simulink model "Oneroom_2015b_Web_Socket"  (R2016a)
settings: Solver=VariableStepAuto  StartTime=0.0  StopTime=Inf  RelTol=1e-3
InitFcn:
  | %server = sim_server(10000);
StartFcn:
  | %The GUI handles are by default hidden, turn them on
  | set(0,'ShowHiddenHandles','on');
  | 
  | %Set up the arguments that will go into the gain block event callback listener
  | blk = 'Oneroom_2015b_Web_Socket/Temperature';
  | event = 'PostOutputs';
  | listener = @updategui;
  | 
  | %Create the listener
  | h = add_exec_event_listener(blk, event, listener);
StopFcn:
  | %server.stop
libraries: simulink x1
settings Model: Creator=accma  LastModifiedBy=e0154145

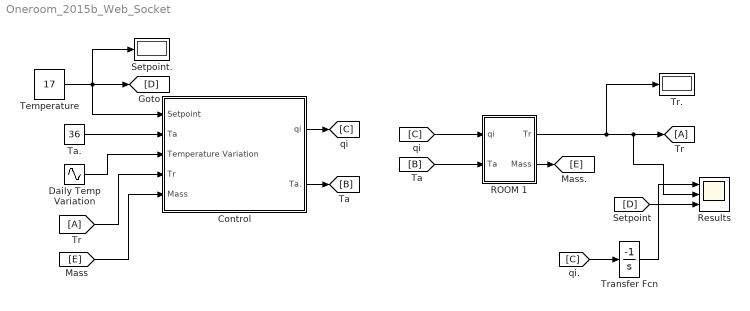
== system Oneroom_2015b_Web_Socket ==
  Control : Subsystem
  Daily Temp Variation : Sin  Amplitude=15  Frequency=2*pi/24  SampleTime=0
  ROOM 1 : Subsystem
  Results : Scope  NumInputPorts=3
  Setpoint. : Display
  Ta. : Constant  Value=36
  Temperature : Constant  Value=17
  Tr. : Display
  Transfer Fcn : TransferFcn  Numerator=[-1]  Denominator=[1 0]
  wires:
  ROOM 1/1(Tr) -> Tr./1, Results/2, [A]
  Ta./1 -> Control/2(Ta)
  Daily Temp Variation/1 -> Control/3(Temperature Variation)
  [B] -> ROOM 1/2(Ta)
  Control/1(qi) -> [C]
  [C] -> ROOM 1/1(qi)
  Control/2(Ta.) -> [B]
  [E] -> Control/5(Mass)
  ROOM 1/2("Mass ") -> [E]
  [A] -> Control/4(Tr)
  [C] -> Transfer Fcn/1
  Transfer Fcn/1 -> Results/1
  [D] -> Results/3
  Temperature/1 -> Control/1(Setpoint), Setpoint./1, [D]

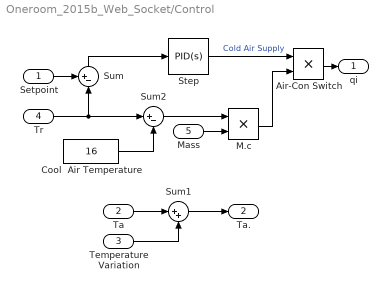
== system Oneroom_2015b_Web_Socket/Control ==
  Setpoint : Inport
  Ta : Inport  Port=2
  Temperature Variation : Inport  Port=3
  Tr : Inport  Port=4
  Mass : Inport  Port=5
  Air-Con Switch : Product  OutMin=16  OutMax=24  RndMeth=Zero
  Cool  Air Temperature : Constant  Value=16
  M.c : Product  RndMeth=Zero
  "Step " : simulink/Continuous/PID Controller  Controller=PID  TimeDomain=Continuous-time  SampleTime=-1  IntegratorMethod=Forward Euler  FilterMethod=Forward Euler  Form=Parallel  UseFilter=on  ControllerParametersSource=internal  P=0.180562771706717  I=1.39450145257241  D=0.00209626055389064  N=23.2260724094918  InitialConditionSource=internal  InitialConditionForIntegrator=0  InitialConditionForFilter=0  ExternalReset=none  LimitOutput=on  UpperSaturationLimit=1  LowerSaturationLimit=-1  LinearizeAsGain=on  AntiWindupMode=none  Kb=1  TrackingMode=off  Kt=1  PParamMin=[]  PParamMax=[]  IParamMin=[]  IParamMax=[]  DParamMin=[]  DParamMax=[]  NParamMin=[]  NParamMax=[]  KbParamMin=[]  KbParamMax=[]  KtParamMin=[]  KtParamMax=[]  POutMin=[]  POutMax=[]  IOutMin=[]  IOutMax=[]  DOutMin=[]  DOutMax=[]  NOutMin=[]  NOutMax=[]  KbOutMin=[]  KbOutMax=[]  KtOutMin=[]  KtOutMax=[]  IntegratorOutMin=[]  IntegratorOutMax=[]  FilterOutMin=[]  FilterOutMax=[]  SumOutMin=[]  SumOutMax=[]  SumI1OutMin=[]  SumI1OutMax=[]  SumI2OutMin=[]  SumI2OutMax=[]  SumI3OutMin=[]  SumI3OutMax=[]  SumDOutMin=[]  SumDOutMax=[]  SaturationOutMin=[]  SaturationOutMax=[]  IntegratorContinuousStateAttributes=''  IntegratorStateMustResolveToSignalObject=off  IntegratorRTWStateStorageClass=Auto  FilterContinuousStateAttributes=''  FilterStateMustResolveToSignalObject=off  FilterRTWStateStorageClass=Auto  DifferentiatorICPrevScaledInput=0  DifferentiatorOutMin=[]  DifferentiatorOutMax=[]
  Sum : Sum  Inputs=+-|  SaturateOnIntegerOverflow=on  InputSameDT=on  OutDataTypeStr=Inherit: Same as first input
  Sum1 : Sum  Inputs=|++  SaturateOnIntegerOverflow=on  InputSameDT=on  OutDataTypeStr=Inherit: Same as first input
  Sum2 : Sum  Inputs=|+-
  qi : Outport
  Ta. : Outport  Port=2
  wires:
  Air-Con Switch/1 -> qi/1
  Ta/1 -> Sum1/1
  Sum1/1 -> Ta./1
  Cool  Air Temperature/1 -> Sum2/2
  Sum/1 -> "Step "/1
  Temperature Variation/1 -> Sum1/2
  Setpoint/1 -> Sum/1
  "Step "/1 -> Air-Con Switch/1  "Cold Air Supply"
  M.c/1 -> Air-Con Switch/2
  Tr/1 -> Sum2/1, Sum/2
  Mass/1 -> M.c/2
  Sum2/1 -> M.c/1

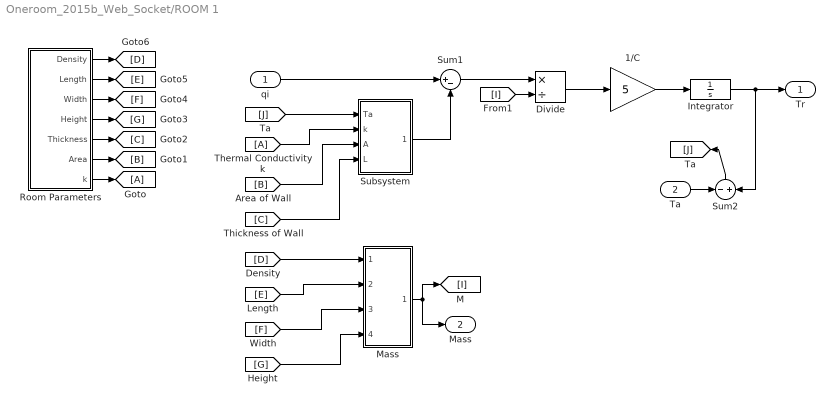
== system Oneroom_2015b_Web_Socket/ROOM 1 ==
  qi : Inport
  Ta : Inport  Port=2
  1/C : Gain  Gain=5  SaturateOnIntegerOverflow=on  OutDataTypeStr=Inherit: Same as input  ParamDataTypeStr=Inherit: Same as input
  Divide : Product  Inputs=*/
  Integrator : Integrator  InitialCondition=30  LimitOutput=on  UpperSaturationLimit=100  LowerSaturationLimit=14
  Mass : Subsystem
  Room Parameters : Subsystem
  Subsystem : Subsystem
  Sum1 : Sum  Inputs=|+-  SaturateOnIntegerOverflow=on  InputSameDT=on  OutDataTypeStr=Inherit: Same as first input
  Sum2 : Sum  Inputs=-+  SaturateOnIntegerOverflow=on  InputSameDT=on  OutDataTypeStr=Inherit: Same as first input
  Tr : Outport  InitialOutput=0
  "Mass " : Outport  Port=2  InitialOutput=0
  wires:
  Divide/1 -> 1/C/1
  Sum1/1 -> Divide/1
  qi/1 -> Sum1/1
  Room Parameters/7(k) -> [A]
  Room Parameters/6("Area ") -> [B]
  Room Parameters/5(Thickness) -> [C]
  Room Parameters/1("Density ") -> [D]
  Room Parameters/2("Length ") -> [E]
  Room Parameters/3("Width ") -> [F]
  Room Parameters/4("Height ") -> [G]
  [J] -> Subsystem/1(Ta)
  [A] -> Subsystem/2(k)
  [B] -> Subsystem/3(A)
  [C] -> Subsystem/4(L)
  Subsystem/1("Ta*kA/L ") -> Sum1/2
  [D] -> Mass/1(Density)
  [E] -> Mass/2(Length)
  [F] -> Mass/3(Width)
  [G] -> Mass/4(Height)
  Integrator/1 -> Tr/1, Sum2/2
  1/C/1 -> Integrator/1
  Mass/1(Mass.) -> [I], "Mass "/1
  [I] -> Divide/2
  Ta/1 -> Sum2/1
  Sum2/1 -> [J]

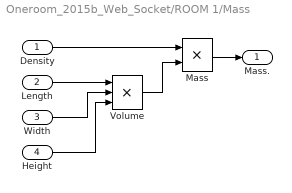
== system Oneroom_2015b_Web_Socket/ROOM 1/Mass ==
  Density : Inport
  Length : Inport  Port=2
  Width : Inport  Port=3
  Height : Inport  Port=4
  Mass : Product
  Volume : Product  Inputs=3
  Mass. : Outport
  wires:
  Volume/1 -> Mass/2
  Density/1 -> Mass/1
  Mass/1 -> Mass./1
  Length/1 -> Volume/1
  Width/1 -> Volume/2
  Height/1 -> Volume/3

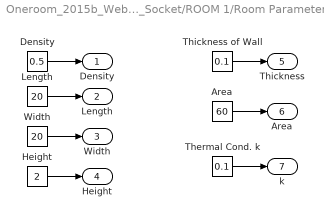
== system Oneroom_2015b_Web_Socket/ROOM 1/Room Parameters ==
  Area : Constant  Value=60
  Density : Constant  Value=0.5
  Height : Constant  Value=2
  Length : Constant  Value=20
  Thermal Cond. k : Constant  Value=0.1
  Thickness of Wall : Constant  Value=0.1
  Width : Constant  Value=20
  "Density " : Outport  InitialOutput=0
  "Length " : Outport  Port=2  InitialOutput=0
  "Width " : Outport  Port=3  InitialOutput=0
  "Height " : Outport  Port=4  InitialOutput=0
  Thickness : Outport  Port=5  InitialOutput=0
  "Area " : Outport  Port=6  InitialOutput=0
  k : Outport  Port=7  InitialOutput=0
  wires:
  Thermal Cond. k/1 -> k/1
  Density/1 -> "Density "/1
  Area/1 -> "Area "/1
  Height/1 -> "Height "/1
  Width/1 -> "Width "/1
  Length/1 -> "Length "/1
  Thickness of Wall/1 -> Thickness/1

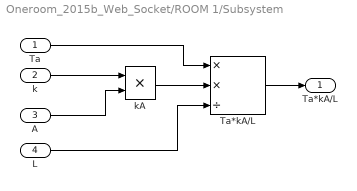
== system Oneroom_2015b_Web_Socket/ROOM 1/Subsystem ==
  Ta : Inport
  k : Inport  Port=2
  A : Inport  Port=3
  L : Inport  Port=4
  Ta*kA/L : Product  Inputs=**/
  kA : Product
  "Ta*kA/L " : Outport
  wires:
  k/1 -> kA/1
  kA/1 -> Ta*kA/L/2
  Ta*kA/L/1 -> "Ta*kA/L "/1
  L/1 -> Ta*kA/L/3
  A/1 -> kA/2
  Ta/1 -> Ta*kA/L/1
